simulink model "reichardt_array_EMD_2"  (R2019a)
settings: Solver=ode45  StartTime=0.0  StopTime=setStopTime  FixedStep=0.0005  RelTol=1e-3  EnableMultiTasking=on
model workspace (MAT data in the model file):
  bodyAmp = 0
  bodyPhase = 0
  freq = 2.96243790602
  headAmp = 0
  headPhase = 0
  imageData = [0.00228480667088 0.00685422825671 0.0114230745906 0.0159909622235 0.0205575077854 0.0251223280162 0.0296850397975 0.0342452601838 0.0388026064343 0.0433566960441 0.0479071467754 0.0524535766893 ... (8204 elements, 1x8204)]
  outputTimeList = [2.12095088792 2.1421603968 2.16336990568 2.18457941456 2.20578892344 2.22699843232 2.2482079412 2.26941745007 2.29062695895 2.31183646783 2.33304597671 2.35425548559 ... (101 elements, 1x101)]
  setStopTime = 4.24190177584
  stimAmp = 15
  temporalFilt = 60
  timeConstant = 0.035
libraries: visionsources x1
(part 2 of 2)

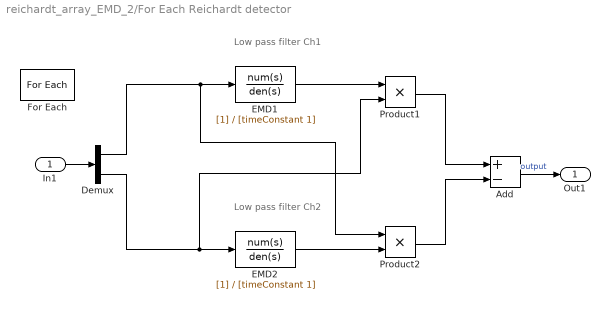
== system reichardt_array_EMD_2/For Each Reichardt detector ==
  note: Low pass filter
      | Ch1
  note: Low pass filter
      | Ch2
  In1 : Inport  Partition=on  PartitionDimension=1  PartitionWidth=1  PartitionOffset=0
  Add : Sum  Inputs=+-
  Demux : Demux  Outputs=2
  EMD1 : TransferFcn  Denominator=[timeConstant 1]
  EMD2 : TransferFcn  Denominator=[timeConstant 1]
  For Each : ForEach  DisableCoverage=on  IndexMode=One-based
  Product1 : Product  RndMeth=Zero
  Product2 : Product  RndMeth=Zero
  Out1 : Outport  ConcatenationDimension=1
  wires:
  EMD1/1 -> Product1/1
  Product1/1 -> Add/1
  Product2/1 -> Add/2
  EMD2/1 -> Product2/2
  Add/1 -> Out1/1  "output"
  In1/1 -> Demux/1
  Demux/1 -> Product2/1, EMD1/1
  Demux/2 -> Product1/2, EMD2/1

== matlab function reichardt_array_EMD_2/sampleImage ==
  data: imageData input; intensity output double size=360,2; seenAngle input
function intensity = fcn(imageData,seenAngle)
%#codegen

imageWidth = length(imageData);

% Subsample with resolution of compound eye
sampleCoord = 0:359;
sampleCoord = sampleCoord + seenAngle;
sampleCoord = mod(sampleCoord,360);
temp        = interp1(linspace(0,360,imageWidth),imageData,sampleCoord);

% Create output signals
intensity = [temp(:), circshift(temp(:),-1)];
